simulink model "Group_HW3_Simulink"  (R2020b)
settings: Solver=VariableStepAuto  StartTime=0.0  StopTime=tstop  RelTol=1e-9
undefined symbols (not defined in the file): cutoff_time, DenPoly, input_select
settings Model: Creator=domin  LastModifiedBy=domin

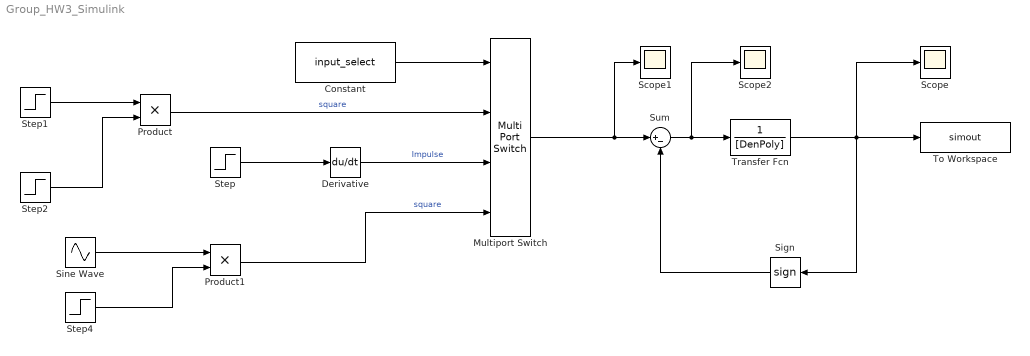
== system Group_HW3_Simulink ==
  Constant : Constant  Value=input_select
  Derivative : Derivative
  Multiport Switch : MultiPortSwitch
  Product : Product
  Product1 : Product
  Scope : Scope
  Scope1 : Scope
  Scope2 : Scope
  Sign : Signum
  Sine Wave : Sin  Amplitude=10^-23  Frequency=2*pi*10^7  SampleTime=0
  Step : Step  Time=10*pi/(10^7)/10  SampleTime=0
  Step1 : Step  Time=pi/(10^7)/10  After=.01  SampleTime=0
  Step2 : Step  Time=cutoff_time  Before=1  After=0  SampleTime=0
  Step4 : Step  Time=cutoff_time  Before=1  After=0  SampleTime=0
  Sum : Sum  Inputs=|+-
  To Workspace : ToWorkspace  VariableName=simout  SaveFormat=Timeseries  SampleTime=-1
  Transfer Fcn : TransferFcn  Denominator=[DenPoly]
  wires:
  Sum/1 -> Scope2/1, Transfer Fcn/1
  Step/1 -> Derivative/1
  Step1/1 -> Product/1
  Step2/1 -> Product/2
  Constant/1 -> Multiport Switch/1
  Product/1 -> Multiport Switch/2  "square"
  Derivative/1 -> Multiport Switch/3  "Impulse"
  Step4/1 -> Product1/2
  Sine Wave/1 -> Product1/1
  Product1/1 -> Multiport Switch/4  "square"
  Multiport Switch/1 -> Scope1/1, Sum/1
  Transfer Fcn/1 -> Sign/1, Scope/1, To Workspace/1
  Sign/1 -> Sum/2
